simulink model "LVS_model_upgrade_OLD"  (R2021a)
settings: Solver=VariableStepAuto  StartTime=0.0  StopTime=80  RelTol=1e-3
values from neighbouring files (symbols this model uses):
  landmarks_initial = zeros(1, landmarks_number_lvs*10+1)    [mc_light.m]    (also in scenario_settings.m)
  Tl = 0.1    [main.m]    (also in mc_light.m)
settings Model: Creator=alber  LastModifiedBy=Paolo.Martella

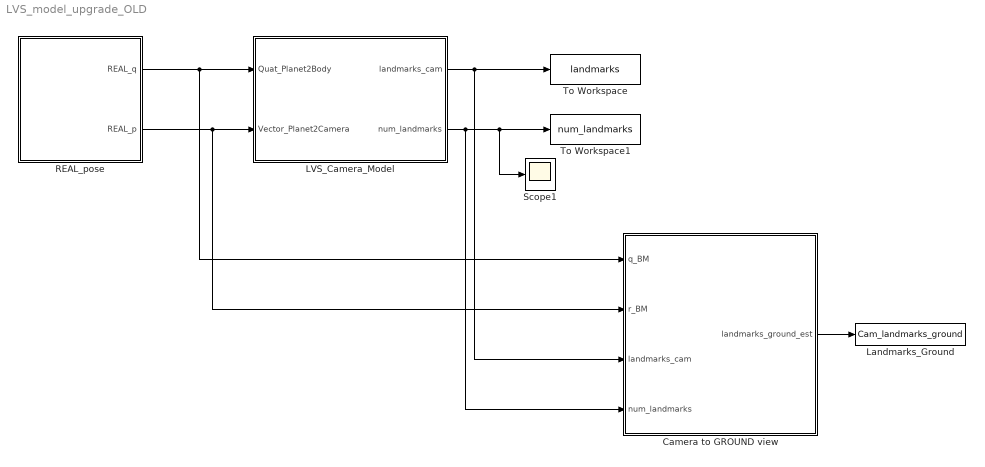
== system LVS_model_upgrade_OLD ==
  Camera to GROUND view : Subsystem
  LVS_Camera_Model : Subsystem
  Landmarks_Ground : ToWorkspace  VariableName=Cam_landmarks_ground  SampleTime=-1
  REAL_pose : Subsystem
  Scope1 : Scope
  To Workspace : ToWorkspace  VariableName=landmarks  SaveFormat=Timeseries  SampleTime=-1
  To Workspace1 : ToWorkspace  VariableName=num_landmarks  SampleTime=-1
  wires:
  REAL_pose/1(REAL_q) -> Camera to GROUND view/1(q_BM), LVS_Camera_Model/1(Quat_Planet2Body)
  LVS_Camera_Model/1(landmarks_cam) -> Camera to GROUND view/3(landmarks_cam), To Workspace/1
  LVS_Camera_Model/2(num_landmarks) -> Camera to GROUND view/4(num_landmarks), Scope1/1, To Workspace1/1
  REAL_pose/2(REAL_p) -> Camera to GROUND view/2(r_BM), LVS_Camera_Model/2(Vector_Planet2Camera)
  Camera to GROUND view/1(landmarks_ground_est) -> Landmarks_Ground/1

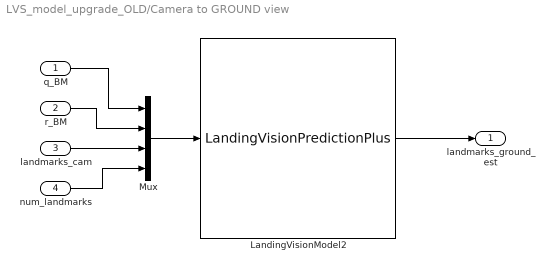
== system LVS_model_upgrade_OLD/Camera to GROUND view ==
  q_BM : Inport
  r_BM : Inport  Port=2
  landmarks_cam : Inport  Port=3
  num_landmarks : Inport  Port=4
  LandingVisionModel2 : S-Function  FunctionName=LandingVisionPredictionPlus  Parameters=-1, r_CB, q_CB, w, h, actualf, n_points  SFunctionDeploymentMode=off  EnableBusSupport=off
  Mux : Mux
  landmarks_ground_est : Outport
  wires:
  landmarks_cam/1 -> Mux/3
  Mux/1 -> LandingVisionModel2/1
  LandingVisionModel2/1 -> landmarks_ground_est/1
  r_BM/1 -> Mux/2
  num_landmarks/1 -> Mux/4
  q_BM/1 -> Mux/1

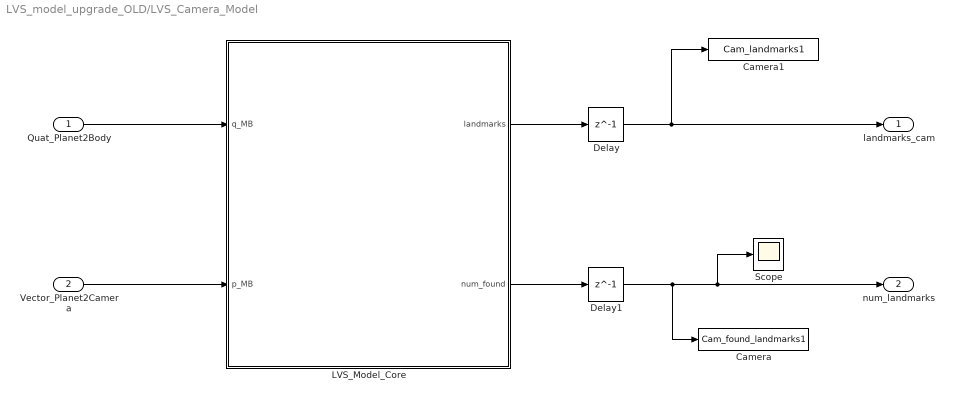
== system LVS_model_upgrade_OLD/LVS_Camera_Model ==
  Quat_Planet2Body : Inport
  Vector_Planet2Camera : Inport  Port=2
  Camera : ToWorkspace  VariableName=Cam_found_landmarks1  SampleTime=-1
  Camera1 : ToWorkspace  VariableName=Cam_landmarks1  SampleTime=-1
  Delay : Delay  DelayLength=1  InitialCondition=landmarks_initial  SampleTime=Tl
  Delay1 : Delay  DelayLength=1  InitialCondition=0  SampleTime=Tl
  LVS_Model_Core : Subsystem
  Scope : Scope
  landmarks_cam : Outport
  num_landmarks : Outport  Port=2
  wires:
  Delay1/1 -> Camera/1, num_landmarks/1, Scope/1
  LVS_Model_Core/1(landmarks) -> Delay/1
  Vector_Planet2Camera/1 -> LVS_Model_Core/2(p_MB)
  Delay/1 -> landmarks_cam/1, Camera1/1
  LVS_Model_Core/2(num_found) -> Delay1/1
  Quat_Planet2Body/1 -> LVS_Model_Core/1(q_MB)

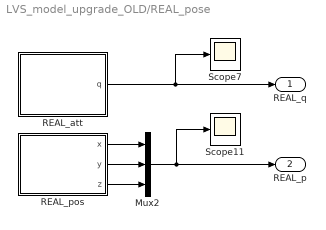
== system LVS_model_upgrade_OLD/REAL_pose ==
  Mux2 : Mux  Inputs=3
  REAL_att : Subsystem
  REAL_pos : Subsystem
  Scope11 : Scope
  Scope7 : Scope
  REAL_q : Outport
  REAL_p : Outport  Port=2
  wires:
  REAL_att/1(q) -> REAL_q/1, Scope7/1
  Mux2/1 -> REAL_p/1, Scope11/1
  REAL_pos/3(z) -> Mux2/3
  REAL_pos/1(x) -> Mux2/1
  REAL_pos/2(y) -> Mux2/2

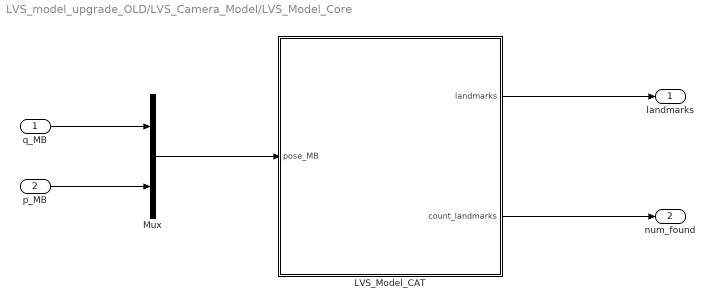
== system LVS_model_upgrade_OLD/LVS_Camera_Model/LVS_Model_Core ==
  q_MB : Inport
  p_MB : Inport  Port=2
  LVS_Model_CAT : Subsystem
  Mux : Mux  Inputs=2
  landmarks : Outport
  num_found : Outport  Port=2
  wires:
  LVS_Model_CAT/2(count_landmarks) -> num_found/1
  LVS_Model_CAT/1(landmarks) -> landmarks/1
  Mux/1 -> LVS_Model_CAT/1(pose_MB)
  q_MB/1 -> Mux/1
  p_MB/1 -> Mux/2

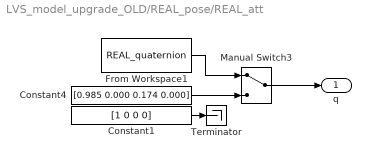
== system LVS_model_upgrade_OLD/REAL_pose/REAL_att ==
  Constant1 : Constant  Value=[1 0 0 0]
  Constant4 : Constant  Value=[0.985 0.000 0.174 0.000]
  From Workspace1 : FromWorkspace  VariableName=REAL_quaternion
  Manual Switch3 : ManualSwitch
  Terminator : Terminator
  q : Outport
  wires:
  Constant1/1 -> Terminator/1
  Manual Switch3/1 -> q/1
  Constant4/1 -> Manual Switch3/2
  From Workspace1/1 -> Manual Switch3/1

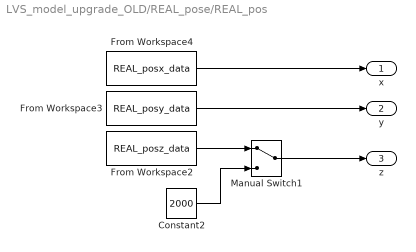
== system LVS_model_upgrade_OLD/REAL_pose/REAL_pos ==
  Constant2 : Constant  Value=2000
  From Workspace2 : FromWorkspace  VariableName=REAL_posz_data
  From Workspace3 : FromWorkspace  VariableName=REAL_posy_data
  From Workspace4 : FromWorkspace  VariableName=REAL_posx_data
  Manual Switch1 : ManualSwitch
  x : Outport
  y : Outport  Port=2
  z : Outport  Port=3
  wires:
  From Workspace2/1 -> Manual Switch1/1
  Manual Switch1/1 -> z/1
  From Workspace3/1 -> y/1
  Constant2/1 -> Manual Switch1/2
  From Workspace4/1 -> x/1

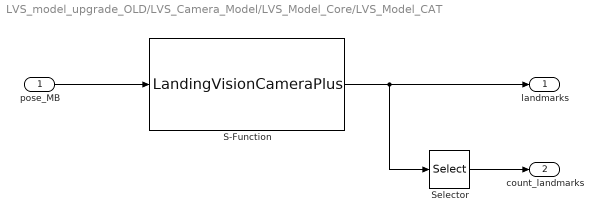
== system LVS_model_upgrade_OLD/LVS_Camera_Model/LVS_Model_Core/LVS_Model_CAT ==
  pose_MB : Inport
  S-Function : S-Function  FunctionName=LandingVisionCameraPlus  Parameters=Tl, Cat, r_CB, q_CB, w, h, actualf, n_points  SFunctionDeploymentMode=off  EnableBusSupport=off
  Selector : Selector  InputPortWidth=1001  IndexOptions=Index vector (dialog)  Indices=[201]  OutputSizes=1
  landmarks : Outport
  count_landmarks : Outport  Port=2
  wires:
  Selector/1 -> count_landmarks/1
  S-Function/1 -> Selector/1, landmarks/1
  pose_MB/1 -> S-Function/1
